simulink model "METI_TM_PNT"  (R2018b)
settings: Solver=ode8  StartTime=0  StopTime=end_time  FixedStep=sampling_time  RelTol=1e-3
PreLoadFcn:
  | METI_TM_PNT_PreLoad;
values from neighbouring files (symbols this model uses):
  sampling_time = 0.0025    [METI_CVT_Slct.m]
undefined symbols (not defined in the file or in its folder): DF_PNT_DF_gear, DF_PNT_Driveshaft_damper, DF_PNT_Driveshaft_delta_radps_LL, DF_PNT_Driveshaft_delta_radps_UL, DF_PNT_Driveshaft_spring, DF_PNT_eta_DF, K2degC, magnitude, radpsec2rpm, TM_PNT_ConvUnit, TM_PNT_Driveshaft_Inertia_kgm2, TM_PNT_eta_CVT, TM_PNT_eta_CVT_x_CVTF_degC, TM_PNT_Flywheel_Inertia_kgm2, TM_PNT_Flywheel_Init_radps, TM_PNT_Gain_LU_damper_Nmsprad, TM_PNT_Gain_LU_spring_Nmprad, TM_PNT_n_TC_min_rpm, TM_PNT_ratio_w_ROT_T_C_LL, TM_PNT_ratio_w_ROT_T_C_UL, TM_PNT_Tau_CVT_ratio_s, TM_PNT_tau_LU_Clutch_s, TM_PNT_torque_capacity_Nmprpm2_table, TM_PNT_torque_capacity_Nmprpm2_table_x_speed_ratio, TM_PNT_torque_ratio_table, TM_PNT_torque_ratio_table_x_speed_ratio, TM_PNT_w_ROT_T_C_LL, TM_PNT_w_ROT_T_C_UL
libraries: METI_Lib_vehicle_model x13, simulink x2
settings Model: Creator=nishimura  LastModifiedBy=E00026
settings DataIOCC: LimitDataPoints=on  SaveFormat=Array  SaveOutput=off  InspectSignalLogs=on  SaveTime=off
settings OptimizationCC: BlockReduction=off  BooleanDataType=off  LifeSpan=inf
settings DebuggingCC: SaveWithParameterizedLinksMsg=none  UnderspecifiedInitializationDetection=Classic  MergeDetectMultiDrivingBlocksExec=none  SignalResolutionControl=TryResolveAllWithWarning  StrictBusMsg=ErrorOnBusTreatedAsVector  SFUnexpectedBacktrackingDiag=warning  SFNoUnconditionalDefaultTransitionDiag=warning  SFExecutionAtInitializationDiag=none
settings HardwareCC: ProdBitPerPointer=32  ProdBitPerSizeT=32  ProdBitPerPtrDiffT=32  ProdLargestAtomicFloat=None  ProdIntDivRoundTo=Undefined  ProdEndianess=Unspecified  ProdWordSize=32  ProdHWDeviceType=32-bit Generic  TargetUnknown=on
settings ModelReferenceCC: ModelReferenceNumInstancesAllowed=Single  PropagateSignalLabelsOutOfModel=off
settings SFSimCC: SimUseLocalCustomCode=off
settings RTWCC: RTWUseLocalCustomCode=off
settings CodeAppCC: StateflowObjectComments=on
settings GRTTargetCC: TargetLangStandard=C89/C90 (ANSI)  GeneratePreprocessorConditionals=Disable all
settings ConfigComp: CovMetricSettings=dw  CovHtmlReporting=on  CovSaveCumulativeToWorkspaceVar=on  CovSaveSingleToWorkspaceVar=on  CovExternalEMLEnable=off  CovSFcnEnable=off

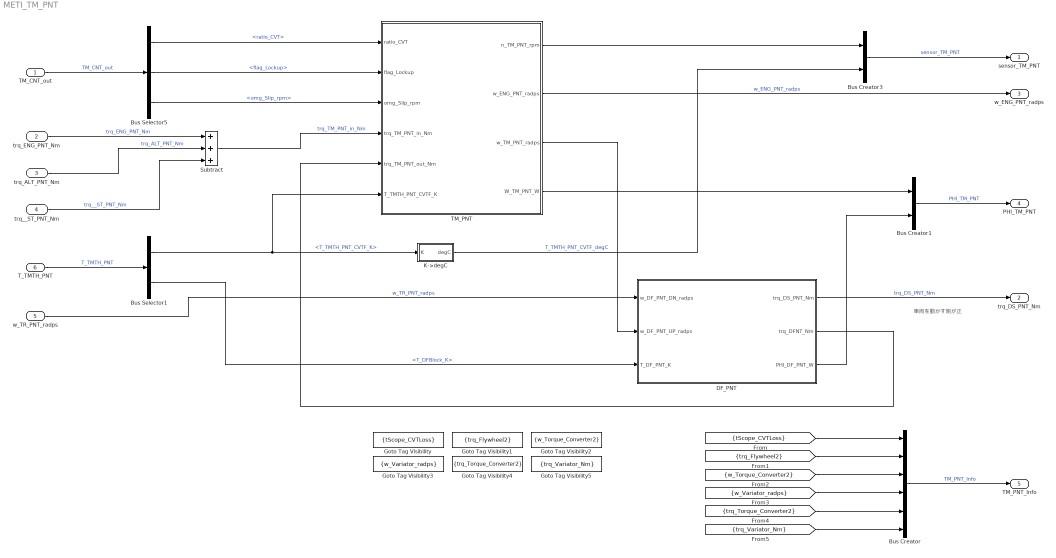
== system METI_TM_PNT ==
  note: 車両を動かす側が正
  TM_CNT_out : Inport  OutDataTypeStr=Bus: TM_CNT_out  SampleTime=sampling_time
      settings: AttributesFormatString=|
      | <SampleTime = %<SampleTime>>
      | <%<OutDataTypeStr>>
  trq_ENG_PNT_Nm : Inport  Port=2  OutDataTypeStr=double  PortDimensions=1  SampleTime=0
      settings: AttributesFormatString=<SampleTime = %<SampleTime>>
  trq_ALT_PNT_Nm : Inport  Port=3  OutDataTypeStr=double  PortDimensions=1  SampleTime=0
      settings: AttributesFormatString=<SampleTime = %<SampleTime>>
  trq__ST_PNT_Nm : Inport  Port=4  OutDataTypeStr=double  PortDimensions=1
      settings: AttributesFormatString=<SampleTime = %<SampleTime>>
  w_TR_PNT_radps : Inport  Port=5  OutDataTypeStr=double  PortDimensions=1  SampleTime=sampling_time
      settings: AttributesFormatString=<SampleTime = %<SampleTime>>
  T_TMTH_PNT : Inport  Port=6  OutDataTypeStr=Bus: T_TMTH_PNT  SampleTime=sampling_time
      settings: AttributesFormatString=|
      | <SampleTime = %<SampleTime>>
      | <%<OutDataTypeStr>>
  Bus Creator : BusCreator  Inputs=6
  Bus Creator1 : BusCreator  Inputs=2
  Bus Creator3 : BusCreator  Inputs=2
  Bus Selector1 : BusSelector  OutputSignals=T_TMTH_PNT_CVTF_K,T_DFBlock_K
  Bus Selector5 : BusSelector  OutputSignals=ratio_CVT,flag_Lockup,omg_Slip_rpm
  DF_PNT : Subsystem
  Goto Tag Visibility : GotoTagVisibility  GotoTag=tScope_CVTLoss
  Goto Tag Visibility1 : GotoTagVisibility  GotoTag=trq_Flywheel2
  Goto Tag Visibility2 : GotoTagVisibility  GotoTag=w_Torque_Converter2
  Goto Tag Visibility3 : GotoTagVisibility  GotoTag=w_Variator_radps
  Goto Tag Visibility4 : GotoTagVisibility  GotoTag=trq_Torque_Converter2
  Goto Tag Visibility5 : GotoTagVisibility  GotoTag=trq_Variator_Nm
  K->degC : Subsystem
  Subtract : Sum  Inputs=3
  TM_PNT : Subsystem
  sensor_TM_PNT : Outport  OutDataTypeStr=Bus: sensor_TM_PNT
      settings: AttributesFormatString=|
      | <SampleTime = %<SampleTime>>
      | <%<OutDataTypeStr>>
  trq_DS_PNT_Nm : Outport  Port=2  OutDataTypeStr=double  PortDimensions=1  SampleTime=0
      settings: AttributesFormatString=<SampleTime = %<SampleTime>>
  w_ENG_PNT_radps : Outport  Port=3  OutDataTypeStr=double  PortDimensions=1  SampleTime=0
      settings: AttributesFormatString=<SampleTime = %<SampleTime>>
  PHI_TM_PNT : Outport  Port=4  OutDataTypeStr=Bus: PHI_TM_PNT  SampleTime=0
      settings: AttributesFormatString=|
      | <SampleTime = %<SampleTime>>
      | <%<OutDataTypeStr>>
  TM_PNT_Info : Outport  Port=5  OutDataTypeStr=Bus: TM_PNT_Info  SampleTime=0
      settings: AttributesFormatString=|
      | <SampleTime = %<SampleTime>>
      | <%<OutDataTypeStr>>
  wires:
  DF_PNT/3(PHI_DF_PNT_W) -> Bus Creator1/2
  TM_PNT/4(W_TM_PNT_W) -> Bus Creator1/1
  Bus Selector5/3 -> TM_PNT/3(omg_Slip_rpm)  "<omg_Slip_rpm>"
  trq_ENG_PNT_Nm/1 -> Subtract/1  "trq_ENG_PNT_Nm"
  Bus Creator3/1 -> sensor_TM_PNT/1  "sensor_TM_PNT"
  trq__ST_PNT_Nm/1 -> Subtract/3  "trq__ST_PNT_Nm"
  TM_PNT/2(w_ENG_PNT_radps) -> w_ENG_PNT_radps/1  "w_ENG_PNT_radps"
  K->degC/1(degC) -> Bus Creator3/2  "T_TMTH_PNT_CVTF_degC"
  Bus Selector5/2 -> TM_PNT/2(flag_Lockup)  "<flag_Lockup>"
  Bus Selector1/1 -> K->degC/1(K), TM_PNT/6(T_TMTH_PNT_CVTF_K)  "<T_TMTH_PNT_CVTF_K>"
  DF_PNT/2(trq_DFNT_Nm) -> TM_PNT/5(trq_TM_PNT_out_Nm)
  Bus Selector5/1 -> TM_PNT/1(ratio_CVT)  "<ratio_CVT>"
  trq_ALT_PNT_Nm/1 -> Subtract/2  "trq_ALT_PNT_Nm"
  TM_PNT/1(n_TM_PNT_rpm) -> Bus Creator3/1
  T_TMTH_PNT/1 -> Bus Selector1/1  "T_TMTH_PNT"
  DF_PNT/1(trq_DS_PNT_Nm) -> trq_DS_PNT_Nm/1  "trq_DS_PNT_Nm"
  TM_PNT/3(w_TM_PNT_radps) -> DF_PNT/2(w_DF_PNT_UP_radps)
  Bus Creator1/1 -> PHI_TM_PNT/1  "PHI_TM_PNT"
  w_TR_PNT_radps/1 -> DF_PNT/1(w_DF_PNT_DN_radps)  "w_TR_PNT_radps"
  Subtract/1 -> TM_PNT/4(trq_TM_PNT_in_Nm)  "trq_TM_PNT_in_Nm"
  Bus Selector1/2 -> DF_PNT/3(T_DF_PNT_K)  "<T_DFBlock_K>"
  TM_CNT_out/1 -> Bus Selector5/1  "TM_CNT_out"
  Bus Creator/1 -> TM_PNT_Info/1  "TM_PNT_Info"
  [tScope_CVTLoss] -> Bus Creator/1
  [trq_Flywheel2] -> Bus Creator/2
  [w_Torque_Converter2] -> Bus Creator/3
  [w_Variator_radps] -> Bus Creator/4
  [trq_Torque_Converter2] -> Bus Creator/5
  [trq_Variator_Nm] -> Bus Creator/6

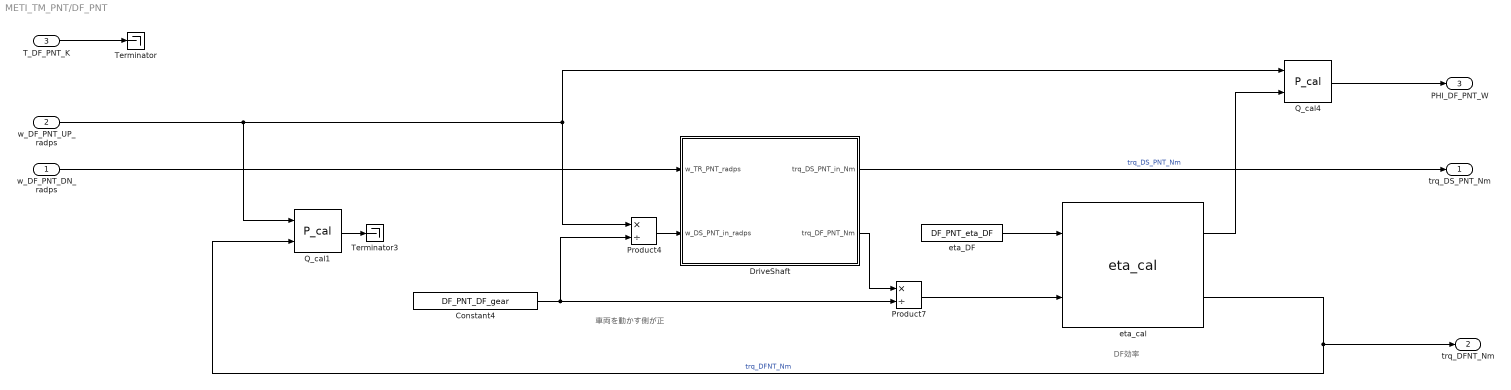
== system METI_TM_PNT/DF_PNT ==
  note: 車両を動かす側が正
  note: DF効率
  w_DF_PNT_DN_radps : Inport
  w_DF_PNT_UP_radps : Inport  Port=2
  T_DF_PNT_K : Inport  Port=3
  Constant4 : Constant  Value=DF_PNT_DF_gear
  DriveShaft : Subsystem
  Product4 : Product  Inputs=*/  RndMeth=Zero
  Product7 : Product  Inputs=*/  RndMeth=Zero
  Q_cal1 : METI_Lib_vehicle_model/P_cal  Type_energy=回転運動  Type_output_energy=出力  Power_name=Po_  t_Workspace_Name=DF_PNT_MECK  P_VariableName=Po_DF_PNT_MECK  Across_VariableName=w_DF_PNT_MECK  Throgh_VariableName=tq_DF_PNT_MECK
  Q_cal4 : METI_Lib_vehicle_model/P_cal  Type_energy=回転運動  Type_output_energy=損失  Power_name=Pl_  t_Workspace_Name=DF_PNT_MECK_LOSS  P_VariableName=Pl_DF_PNT_MECK_LOSS  Across_VariableName=w_DF_PNT_MECK_LOSS  Throgh_VariableName=tq_DF_PNT_MECK_LOSS
  Terminator : Terminator
  Terminator3 : Terminator
  eta_DF : Constant  Value=DF_PNT_eta_DF
  eta_cal : METI_Lib_vehicle_model/eta_cal  SystemSampleTime=-1
  trq_DS_PNT_Nm : Outport
  trq_DFNT_Nm : Outport  Port=2
  PHI_DF_PNT_W : Outport  Port=3
  wires:
  T_DF_PNT_K/1 -> Terminator/1
  Q_cal4/1 -> PHI_DF_PNT_W/1
  DriveShaft/2(trq_DF_PNT_Nm) -> Product7/1
  w_DF_PNT_DN_radps/1 -> DriveShaft/1(w_TR_PNT_radps)
  Product4/1 -> DriveShaft/2(w_DS_PNT_in_radps)
  DriveShaft/1(trq_DS_PNT_in_Nm) -> trq_DS_PNT_Nm/1  "trq_DS_PNT_Nm"
  Product7/1 -> eta_cal/2
  Constant4/1 -> Product4/2, Product7/2
  Q_cal1/1 -> Terminator3/1
  eta_cal/1 -> Q_cal4/2
  eta_cal/2 -> trq_DFNT_Nm/1, Q_cal1/2  "trq_DFNT_Nm"
  eta_DF/1 -> eta_cal/1
  w_DF_PNT_UP_radps/1 -> Q_cal1/1, Q_cal4/1, Product4/1

== system METI_TM_PNT/K->degC ==
  K : Inport
  Constant2 : Constant  Value=K2degC
  Sum : Sum  Inputs=++|
  degC : Outport
  wires:
  Sum/1 -> degC/1
  Constant2/1 -> Sum/1
  K/1 -> Sum/2

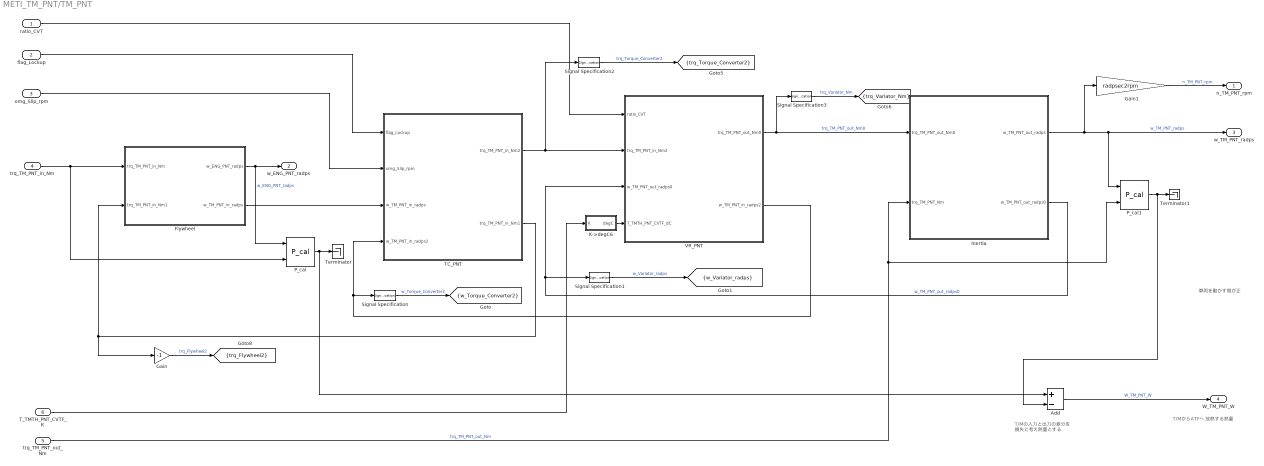
== system METI_TM_PNT/TM_PNT ==
  note: T/Mの入力と出力の差分を
      | 損失と考え熱量とする
  note: T/MからATFへ
      | 放熱する熱量
  note: 車両を動かす側が正
  ratio_CVT : Inport
  flag_Lockup : Inport  Port=2
  omg_Slip_rpm : Inport  Port=3
  trq_TM_PNT_in_Nm : Inport  Port=4
  trq_TM_PNT_out_Nm : Inport  Port=5
  T_TMTH_PNT_CVTF_K : Inport  Port=6
  Add : Sum  Inputs=+-
  Flywheel : Subsystem
  Gain : Gain  Gain=-1
  Gain1 : Gain  Gain=radpsec2rpm
  Inertia : Subsystem
  K->degC6 : Subsystem
  P_cal : METI_Lib_vehicle_model/P_cal  Type_energy=回転運動  Type_output_energy=出力  Power_name=Po_  t_Workspace_Name=TM_PNT_MECK_UP  P_VariableName=Po_TM_PNT_MECK_UP  Across_VariableName=w_TM_PNT_MECK_UP  Throgh_VariableName=tq_TM_PNT_MECK_UP
  P_cal1 : METI_Lib_vehicle_model/P_cal  Type_energy=回転運動  Type_output_energy=出力  Power_name=Po_  t_Workspace_Name=TM_PNT_MECK_DN  P_VariableName=Po_TM_PNT_MECK_DN  Across_VariableName=w_TM_PNT_MECK_DN  Throgh_VariableName=tq_TM_PNT_MECK_DN
  Signal Specification{,1..3} (4 alike) : SignalSpecification
  TC_PNT : Subsystem
  Terminator : Terminator
  Terminator1 : Terminator
  VR_PNT : Subsystem
  n_TM_PNT_rpm : Outport
  w_ENG_PNT_radps : Outport  Port=2
  w_TM_PNT_radps : Outport  Port=3
  W_TM_PNT_W : Outport  Port=4
  tag scope: trq_Flywheel2=scoped, trq_Torque_Converter2=scoped, trq_Variator_Nm=scoped, w_Torque_Converter2=scoped, w_Variator_radps=scoped
  wires:
  Signal Specification3/1 -> [trq_Variator_Nm]  "trq_Variator_Nm"
  Signal Specification2/1 -> [trq_Torque_Converter2]  "trq_Torque_Converter2"
  Signal Specification1/1 -> [w_Variator_radps]  "w_Variator_radps"
  Signal Specification/1 -> [w_Torque_Converter2]  "w_Torque_Converter2"
  K->degC6/1(degC) -> VR_PNT/4(T_TMTH_PNT_CVTF_dC)
  Gain/1 -> [trq_Flywheel2]  "trq_Flywheel2"
  T_TMTH_PNT_CVTF_K/1 -> K->degC6/1(K)
  Add/1 -> W_TM_PNT_W/1  "W_TM_PNT_W"
  VR_PNT/1(trq_TM_PNT_out_Nm0) -> Inertia/1(trq_TM_PNT_out_Nm0), Signal Specification3/1  "trq_TM_PNT_out_Nm0"
  Inertia/2(w_TM_PNT_out_radps0) -> VR_PNT/3(w_TM_PNT_out_radps0), Signal Specification1/1  "w_TM_PNT_out_radps0"
  trq_TM_PNT_out_Nm/1 -> P_cal1/2, Inertia/2(trq_TM_PNT_Nm)  "trq_TM_PNT_out_Nm"
  P_cal1/1 -> Add/2, Terminator1/1
  P_cal/1 -> Terminator/1, Add/1
  Gain1/1 -> n_TM_PNT_rpm/1  "n_TM_PNT_rpm"
  Inertia/1(w_TM_PNT_out_radps) -> Gain1/1, P_cal1/1, w_TM_PNT_radps/1  "w_TM_PNT_radps"
  trq_TM_PNT_in_Nm/1 -> Flywheel/1(trq_TM_PNT_in_Nm), P_cal/2
  Flywheel/1(w_ENG_PNT_radps) -> P_cal/1, w_ENG_PNT_radps/1  "w_ENG_PNT_radps"
  Flywheel/2(w_TM_PNT_in_radps) -> TC_PNT/3(w_TM_PNT_in_radps)
  TC_PNT/2(trq_TM_PNT_in_Nm1) -> Flywheel/2(trq_TM_PNT_in_Nm1), Gain/1
  ratio_CVT/1 -> VR_PNT/1(ratio_CVT)
  omg_Slip_rpm/1 -> TC_PNT/2(omg_Slip_rpm)
  flag_Lockup/1 -> TC_PNT/1(flag_Lockup)
  TC_PNT/1(trq_TM_PNT_in_Nm2) -> VR_PNT/2(trq_TM_PNT_in_Nm2), Signal Specification2/1
  VR_PNT/2(w_TM_PNT_in_radps2) -> TC_PNT/4(w_TM_PNT_in_radps2), Signal Specification/1

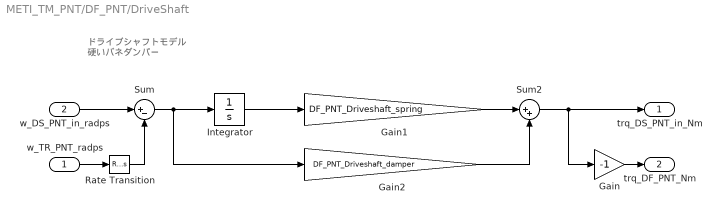
== system METI_TM_PNT/DF_PNT/DriveShaft ==
  note: ドライブシャフトモデル
      | 硬いバネダンパー
  w_TR_PNT_radps : Inport
  w_DS_PNT_in_radps : Inport  Port=2
  Gain : Gain  Gain=-1
  Gain1 : Gain  Gain=DF_PNT_Driveshaft_spring
  Gain2 : Gain  Gain=DF_PNT_Driveshaft_damper
  Integrator : Integrator  LimitOutput=on  UpperSaturationLimit=DF_PNT_Driveshaft_delta_radps_UL  LowerSaturationLimit=DF_PNT_Driveshaft_delta_radps_LL
  Rate Transition : RateTransition  Deterministic=off
  Sum : Sum  Inputs=|+-
  Sum2 : Sum  Inputs=|++
  trq_DS_PNT_in_Nm : Outport
  trq_DF_PNT_Nm : Outport  Port=2
  wires:
  Rate Transition/1 -> Sum/2
  Gain/1 -> trq_DF_PNT_Nm/1
  Sum2/1 -> trq_DS_PNT_in_Nm/1, Gain/1
  Gain2/1 -> Sum2/2
  Gain1/1 -> Sum2/1
  Sum/1 -> Gain2/1, Integrator/1
  Integrator/1 -> Gain1/1
  w_DS_PNT_in_radps/1 -> Sum/1
  w_TR_PNT_radps/1 -> Rate Transition/1

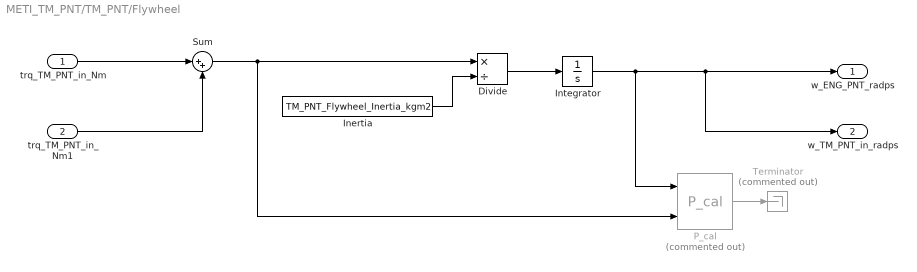
== system METI_TM_PNT/TM_PNT/Flywheel ==
  trq_TM_PNT_in_Nm : Inport
  trq_TM_PNT_in_Nm1 : Inport  Port=2
  Divide : Product  Inputs=*/
  Inertia : Constant  Value=TM_PNT_Flywheel_Inertia_kgm2
  Integrator : Integrator  InitialCondition=TM_PNT_Flywheel_Init_radps  LimitOutput=on  LowerSaturationLimit=0
  P_cal : METI_Lib_vehicle_model/P_cal  Commented=on  Type_energy=回転運動  Type_output_energy=出力  Power_name=Po_  t_Workspace_Name=TM_PNT_Flywheel  P_VariableName=Po_TM_PNT_Flywheel  Across_VariableName=w_TM_PNT_Flywheel  Throgh_VariableName=tq_TM_PNT_Flywheel
  Sum : Sum  Inputs=|++
  Terminator : Terminator  Commented=on
  w_ENG_PNT_radps : Outport
  w_TM_PNT_in_radps : Outport  Port=2
  wires:
  Divide/1 -> Integrator/1
  P_cal/1 -> Terminator/1
  Sum/1 -> P_cal/2, Divide/1
  Inertia/1 -> Divide/2
  trq_TM_PNT_in_Nm1/1 -> Sum/2
  trq_TM_PNT_in_Nm/1 -> Sum/1
  Integrator/1 -> w_ENG_PNT_radps/1, w_TM_PNT_in_radps/1, P_cal/1

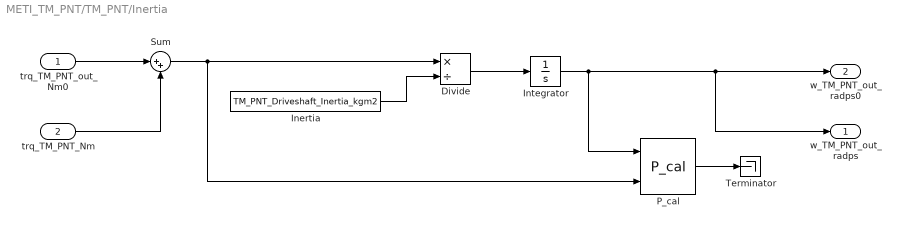
== system METI_TM_PNT/TM_PNT/Inertia ==
  trq_TM_PNT_out_Nm0 : Inport
  trq_TM_PNT_Nm : Inport  Port=2
  Divide : Product  Inputs=*/
  Inertia : Constant  Value=TM_PNT_Driveshaft_Inertia_kgm2
  Integrator : Integrator  InitialCondition=000*(2*pi)/60  LimitOutput=on  LowerSaturationLimit=0
  P_cal : METI_Lib_vehicle_model/P_cal  Type_energy=回転運動  Type_output_energy=出力  Power_name=Po_  t_Workspace_Name=TM_PNT_inertia_MECK  P_VariableName=Po_TM_PNT_inertia_MECK  Across_VariableName=w_TM_PNT_inertia_MECK  Throgh_VariableName=tq_TM_PNT_inertia_MECK
  Sum : Sum  Inputs=|++
  Terminator : Terminator
  w_TM_PNT_out_radps : Outport
  w_TM_PNT_out_radps0 : Outport  Port=2
  wires:
  P_cal/1 -> Terminator/1
  Sum/1 -> P_cal/2, Divide/1
  Inertia/1 -> Divide/2
  trq_TM_PNT_Nm/1 -> Sum/2
  trq_TM_PNT_out_Nm0/1 -> Sum/1
  Divide/1 -> Integrator/1
  Integrator/1 -> w_TM_PNT_out_radps/1, w_TM_PNT_out_radps0/1, P_cal/1

== system METI_TM_PNT/TM_PNT/K->degC6 ==
  K : Inport
  Constant2 : Constant  Value=K2degC
  Sum : Sum  Inputs=++|
  degC : Outport
  wires:
  Sum/1 -> degC/1
  Constant2/1 -> Sum/1
  K/1 -> Sum/2

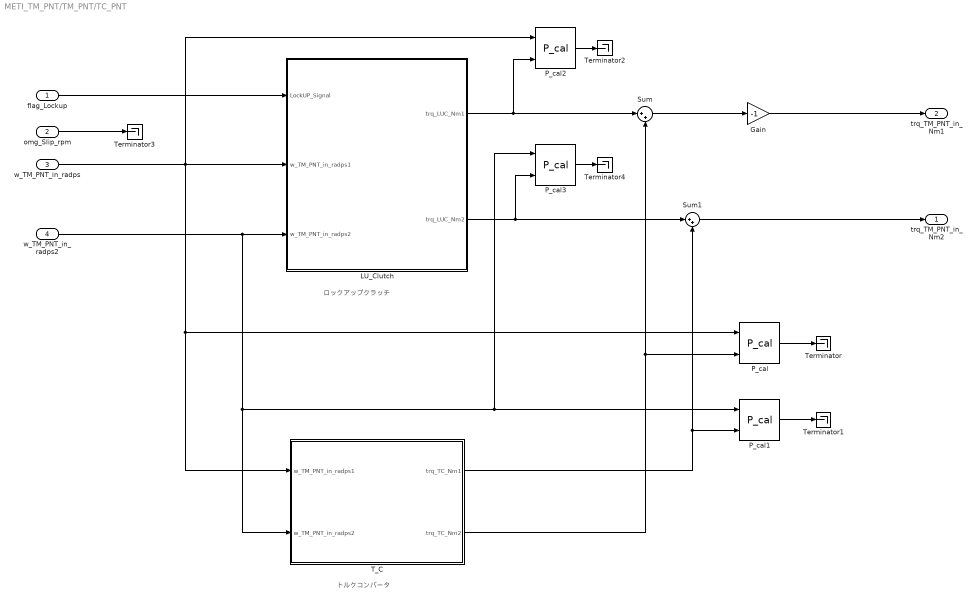
== system METI_TM_PNT/TM_PNT/TC_PNT ==
  note: トルクコンバータ
  note: ロックアップクラッチ
  flag_Lockup : Inport
  omg_Slip_rpm : Inport  Port=2
  w_TM_PNT_in_radps : Inport  Port=3
  w_TM_PNT_in_radps2 : Inport  Port=4
  Gain : Gain  Gain=-1
  LU_Clutch : Subsystem
  P_cal : METI_Lib_vehicle_model/P_cal  Type_energy=回転運動  Type_output_energy=出力  Power_name=Po_  t_Workspace_Name=TM_PNT_TC_MECK_UP  P_VariableName=Po_TM_PNT_TC_MECK_UP  Across_VariableName=w_TM_PNT_TC_MECK_UP  Throgh_VariableName=tq_TM_PNT_TC_MECK_UP
  P_cal1 : METI_Lib_vehicle_model/P_cal  Type_energy=回転運動  Type_output_energy=出力  Power_name=Po_  t_Workspace_Name=TM_PNT_TC_MECK_DN  P_VariableName=Po_TM_PNT_TC_MECK_DN  Across_VariableName=w_TM_PNT_TC_MECK_DN  Throgh_VariableName=tq_TM_PNT_TC_MECK_DN
  P_cal2 : METI_Lib_vehicle_model/P_cal  Type_energy=回転運動  Type_output_energy=出力  Power_name=Po_  t_Workspace_Name=TM_PNT_LU_MECK_UP  P_VariableName=Po_TM_PNT_LU_MECK_UP  Across_VariableName=w_TM_PNT_LU_MECK_UP  Throgh_VariableName=tq_TM_PNT_LU_MECK_UP
  P_cal3 : METI_Lib_vehicle_model/P_cal  Type_energy=回転運動  Type_output_energy=出力  Power_name=Po_  t_Workspace_Name=TM_PNT_LU_MECK_DN  P_VariableName=Po_TM_PNT_LU_MECK_DN  Across_VariableName=w_TM_PNT_LU_MECK_DN  Throgh_VariableName=tq_TM_PNT_LU_MECK_DN
  Sum : Sum  Inputs=|++
  Sum1 : Sum  Inputs=|++
  T_C : Subsystem
  Terminator{,1..4} (5 alike) : Terminator
  trq_TM_PNT_in_Nm2 : Outport
  trq_TM_PNT_in_Nm1 : Outport  Port=2
  wires:
  Gain/1 -> trq_TM_PNT_in_Nm1/1
  P_cal3/1 -> Terminator4/1
  P_cal2/1 -> Terminator2/1
  flag_Lockup/1 -> LU_Clutch/1(LockUP_Signal)
  LU_Clutch/2(trq_LUC_Nm2) -> P_cal3/2, Sum1/1
  LU_Clutch/1(trq_LUC_Nm1) -> P_cal2/2, Sum/1
  omg_Slip_rpm/1 -> Terminator3/1
  P_cal1/1 -> Terminator1/1
  P_cal/1 -> Terminator/1
  w_TM_PNT_in_radps2/1 -> T_C/2(w_TM_PNT_in_radps2), P_cal3/1, P_cal1/1, LU_Clutch/3(w_TM_PNT_in_radps2)
  Sum1/1 -> trq_TM_PNT_in_Nm2/1
  T_C/1(trq_TC_Nm1) -> Sum1/2, P_cal1/2
  Sum/1 -> Gain/1
  w_TM_PNT_in_radps/1 -> P_cal2/1, LU_Clutch/2(w_TM_PNT_in_radps1), P_cal/1, T_C/1(w_TM_PNT_in_radps1)
  T_C/2(trq_TC_Nm2) -> P_cal/2, Sum/2

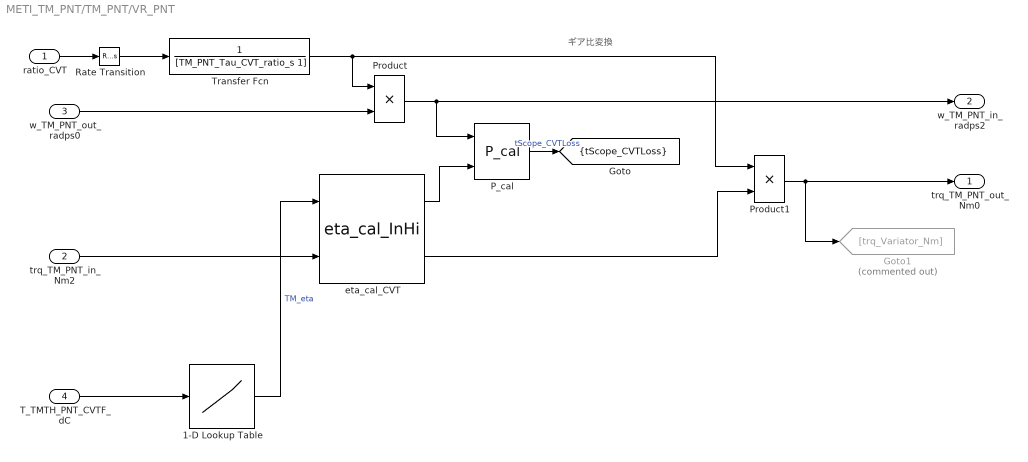
== system METI_TM_PNT/TM_PNT/VR_PNT ==
  note: ギア比変換
  ratio_CVT : Inport
  trq_TM_PNT_in_Nm2 : Inport  Port=2
  w_TM_PNT_out_radps0 : Inport  Port=3
  T_TMTH_PNT_CVTF_dC : Inport  Port=4
  1-D Lookup Table : Lookup_n-D  NumberOfTableDimensions=1  BreakpointsForDimension1=TM_PNT_eta_CVT_x_CVTF_degC  Table=TM_PNT_eta_CVT  ExtrapMethod=Clip  InternalRulePriority=Speed  RndMeth=Simplest  InputSameDT=on
  Goto1 : Goto  Commented=on  GotoTag=trq_Variator_Nm
  P_cal : METI_Lib_vehicle_model/P_cal  Type_energy=回転運動  Type_output_energy=損失  Power_name=Pl_  t_Workspace_Name=TM_PNT_Variator_MECK_LOSS  P_VariableName=Pl_TM_PNT_Variator_MECK_LOSS  Across_VariableName=w_TM_PNT_Variator_MECK_LOSS  Throgh_VariableName=tq_TM_PNT_Variator_MECK_LOSS
  Product : Product  RndMeth=Zero
  Product1 : Product  RndMeth=Zero
  Rate Transition : RateTransition  Deterministic=off
  Transfer Fcn : TransferFcn  Denominator=[TM_PNT_Tau_CVT_ratio_s 1]
  eta_cal_CVT : METI_Lib_vehicle_model/eta_cal_InHi  SystemSampleTime=-1
  trq_TM_PNT_out_Nm0 : Outport
  w_TM_PNT_in_radps2 : Outport  Port=2
  tag scope: tScope_CVTLoss=scoped
  wires:
  Rate Transition/1 -> Transfer Fcn/1
  T_TMTH_PNT_CVTF_dC/1 -> 1-D Lookup Table/1
  eta_cal_CVT/1 -> P_cal/2
  1-D Lookup Table/1 -> eta_cal_CVT/1  "TM_eta"
  Transfer Fcn/1 -> Product/1, Product1/1
  P_cal/1 -> [tScope_CVTLoss]  "tScope_CVTLoss"
  eta_cal_CVT/2 -> Product1/2
  Product1/1 -> trq_TM_PNT_out_Nm0/1, Goto1/1
  ratio_CVT/1 -> Rate Transition/1
  w_TM_PNT_out_radps0/1 -> Product/2
  Product/1 -> P_cal/1, w_TM_PNT_in_radps2/1
  trq_TM_PNT_in_Nm2/1 -> eta_cal_CVT/2

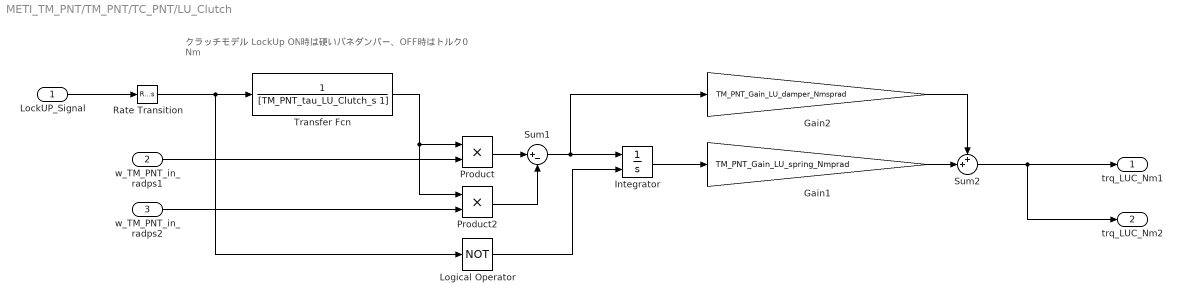
== system METI_TM_PNT/TM_PNT/TC_PNT/LU_Clutch ==
  note: クラッチモデル
      | LockUp ON時は硬いバネダンパー、OFF時はトルク0 Nm
  LockUP_Signal : Inport
  w_TM_PNT_in_radps1 : Inport  Port=2
  w_TM_PNT_in_radps2 : Inport  Port=3
  Gain1 : Gain  Gain=TM_PNT_Gain_LU_spring_Nmprad
  Gain2 : Gain  Gain=TM_PNT_Gain_LU_damper_Nmsprad
  Integrator : Integrator  ExternalReset=level  LimitOutput=on  UpperSaturationLimit=1  LowerSaturationLimit=-1
  Logical Operator : Logic  Operator=NOT  AllPortsSameDT=off  OutDataTypeStr=boolean
  Product : Product  RndMeth=Zero
  Product2 : Product  RndMeth=Zero
  Rate Transition : RateTransition  Deterministic=off
  Sum1 : Sum  Inputs=|+-
  Sum2 : Sum  Inputs=++|
  Transfer Fcn : TransferFcn  Denominator=[TM_PNT_tau_LU_Clutch_s 1]
  trq_LUC_Nm1 : Outport
  trq_LUC_Nm2 : Outport  Port=2
  wires:
  Rate Transition/1 -> Transfer Fcn/1, Logical Operator/1
  Gain2/1 -> Sum2/1
  Gain1/1 -> Sum2/2
  Logical Operator/1 -> Integrator/2
  w_TM_PNT_in_radps2/1 -> Product2/2
  Transfer Fcn/1 -> Product/1, Product2/1
  Sum1/1 -> Gain2/1, Integrator/1
  Integrator/1 -> Gain1/1
  Product/1 -> Sum1/1
  Product2/1 -> Sum1/2
  Sum2/1 -> trq_LUC_Nm1/1, trq_LUC_Nm2/1
  LockUP_Signal/1 -> Rate Transition/1
  w_TM_PNT_in_radps1/1 -> Product/2

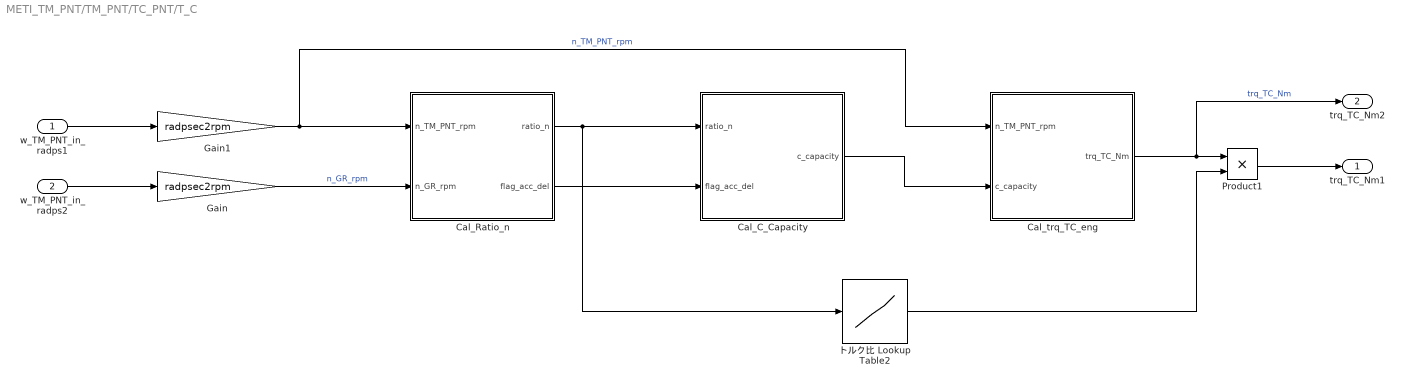
== system METI_TM_PNT/TM_PNT/TC_PNT/T_C ==
  w_TM_PNT_in_radps1 : Inport
  w_TM_PNT_in_radps2 : Inport  Port=2
  Cal_C_Capacity : Subsystem
  Cal_Ratio_n : Subsystem
  Cal_trq_TC_eng : Subsystem
  Gain : Gain  Gain=radpsec2rpm
  Gain1 : Gain  Gain=radpsec2rpm
  Product1 : Product  RndMeth=Zero
  トルク比 Lookup Table2 : Lookup_n-D  NumberOfTableDimensions=1  BreakpointsForDimension1=TM_PNT_torque_ratio_table_x_speed_ratio  Table=TM_PNT_torque_ratio_table  ExtrapMethod=Clip  RndMeth=Simplest  InputSameDT=on
  trq_TC_Nm1 : Outport
  trq_TC_Nm2 : Outport  Port=2
  wires:
  Cal_Ratio_n/2(flag_acc_del) -> Cal_C_Capacity/2(flag_acc_del)
  Cal_C_Capacity/1(c_capacity) -> Cal_trq_TC_eng/2(c_capacity)
  Cal_trq_TC_eng/1(trq_TC_Nm) -> Product1/1, trq_TC_Nm2/1  "trq_TC_Nm"
  Cal_Ratio_n/1(ratio_n) -> Cal_C_Capacity/1(ratio_n), トルク比 Lookup Table2/1
  w_TM_PNT_in_radps1/1 -> Gain1/1
  トルク比 Lookup Table2/1 -> Product1/2
  Product1/1 -> trq_TC_Nm1/1
  w_TM_PNT_in_radps2/1 -> Gain/1
  Gain1/1 -> Cal_trq_TC_eng/1("n_TM_PNT_rpm "), Cal_Ratio_n/1(n_TM_PNT_rpm)  "n_TM_PNT_rpm"
  Gain/1 -> Cal_Ratio_n/2(n_GR_rpm)  "n_GR_rpm"

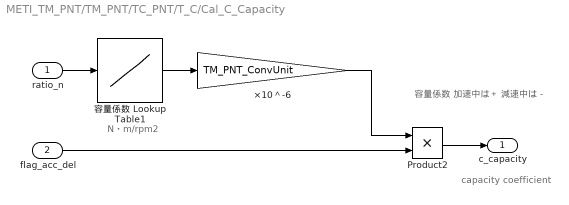
== system METI_TM_PNT/TM_PNT/TC_PNT/T_C/Cal_C_Capacity ==
  note: N・m/rpm2
  note: capacity coefficient
  note: 容量係数
      | 加速中は＋
      | 減速中は－
  ratio_n : Inport
  flag_acc_del : Inport  Port=2
  Product2 : Product  RndMeth=Zero
  ×10＾-6 : Gain  Gain=TM_PNT_ConvUnit
  容量係数 Lookup Table1 : Lookup_n-D  NumberOfTableDimensions=1  BreakpointsForDimension1=TM_PNT_torque_capacity_Nmprpm2_table_x_speed_ratio  Table=TM_PNT_torque_capacity_Nmprpm2_table  RndMeth=Simplest  InputSameDT=on
  c_capacity : Outport
  wires:
  flag_acc_del/1 -> Product2/2
  Product2/1 -> c_capacity/1
  ratio_n/1 -> 容量係数 Lookup Table1/1
  ×10＾-6/1 -> Product2/1
  容量係数 Lookup Table1/1 -> ×10＾-6/1

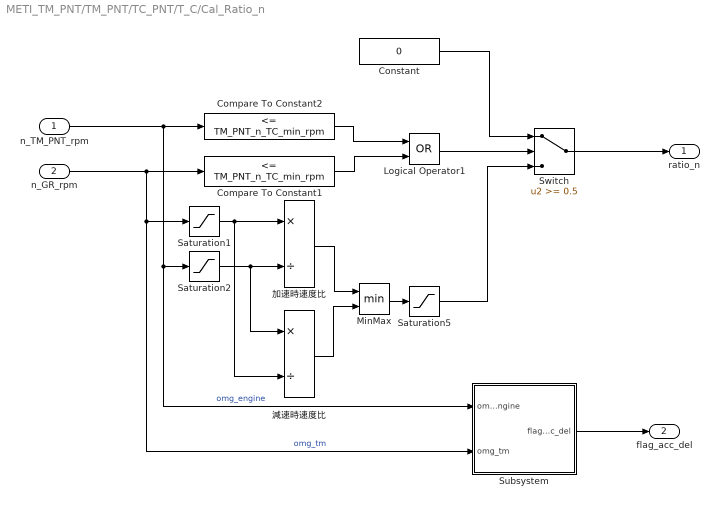
== system METI_TM_PNT/TM_PNT/TC_PNT/T_C/Cal_Ratio_n ==
  n_TM_PNT_rpm : Inport
  n_GR_rpm : Inport  Port=2
  Compare To Constant1 : simulink/Logic and Bit Operations/Compare To Constant  relop=<=  const=TM_PNT_n_TC_min_rpm  OutDataTypeStr=boolean
  Compare To Constant2 : simulink/Logic and Bit Operations/Compare To Constant  relop=<=  const=TM_PNT_n_TC_min_rpm  OutDataTypeStr=boolean
  Constant : Constant  Value=0
  Logical Operator1 : Logic  Operator=OR  AllPortsSameDT=off  OutDataTypeStr=boolean
  MinMax : MinMax  Inputs=2
  Saturation1 : Saturate  UpperLimit=TM_PNT_w_ROT_T_C_UL  LowerLimit=TM_PNT_w_ROT_T_C_LL
  Saturation2 : Saturate  UpperLimit=TM_PNT_w_ROT_T_C_UL  LowerLimit=TM_PNT_w_ROT_T_C_LL
  Saturation5 : Saturate  UpperLimit=TM_PNT_ratio_w_ROT_T_C_UL  LowerLimit=TM_PNT_ratio_w_ROT_T_C_LL
  Subsystem : Subsystem
  Switch : Switch  Threshold=0.5
  加速時速度比 : Product  Inputs=*/
  減速時速度比 : Product  Inputs=*/
  ratio_n : Outport
  flag_acc_del : Outport  Port=2
  wires:
  Subsystem/1(flag_acc_del) -> flag_acc_del/1
  n_TM_PNT_rpm/1 -> Saturation2/1, Subsystem/1(omg_engine), Compare To Constant2/1  "omg_engine"
  n_GR_rpm/1 -> Compare To Constant1/1, Saturation1/1, Subsystem/2(omg_tm)  "omg_tm"
  Switch/1 -> ratio_n/1
  Logical Operator1/1 -> Switch/2
  Compare To Constant1/1 -> Logical Operator1/2
  Compare To Constant2/1 -> Logical Operator1/1
  Constant/1 -> Switch/1
  Saturation5/1 -> Switch/3
  MinMax/1 -> Saturation5/1
  減速時速度比/1 -> MinMax/2
  加速時速度比/1 -> MinMax/1
  Saturation1/1 -> 加速時速度比/1, 減速時速度比/2
  Saturation2/1 -> 加速時速度比/2, 減速時速度比/1

== system METI_TM_PNT/TM_PNT/TC_PNT/T_C/Cal_trq_TC_eng ==
  "n_TM_PNT_rpm " : Inport
  c_capacity : Inport  Port=2
  Math Function : Math  Operator=magnitude^2  SaturateOnIntegerOverflow=on
  Product : Product  RndMeth=Zero
  trq_TC_Nm : Outport
  wires:
  "n_TM_PNT_rpm "/1 -> Math Function/1
  c_capacity/1 -> Product/2
  Math Function/1 -> Product/1
  Product/1 -> trq_TC_Nm/1

== system METI_TM_PNT/TM_PNT/TC_PNT/T_C/Cal_Ratio_n/Subsystem ==
  note: エンジン加速中は1、減速中は-1
  omg_engine : Inport
  omg_tm : Inport  Port=2
  Saturation : Saturate  UpperLimit=1  LowerLimit=-1
  Subtract : Sum  Inputs=-+|
  flag_acc_del : Outport
  wires:
  omg_engine/1 -> Subtract/2
  omg_tm/1 -> Subtract/1
  Saturation/1 -> flag_acc_del/1
  Subtract/1 -> Saturation/1
